simulink model "test_conv2drelu"  (R2017a)
settings: Solver=FixedStepDiscrete  StartTime=0.0  StopTime=1  FixedStep=1  RelTol=1e-3
undefined symbols (not defined in the file or in its folder): gray
libraries: ad_blocks x8, visionsources x1, visiongeotforms x1
settings Model: Creator=eruffaldi  LastModifiedBy=eruffaldi

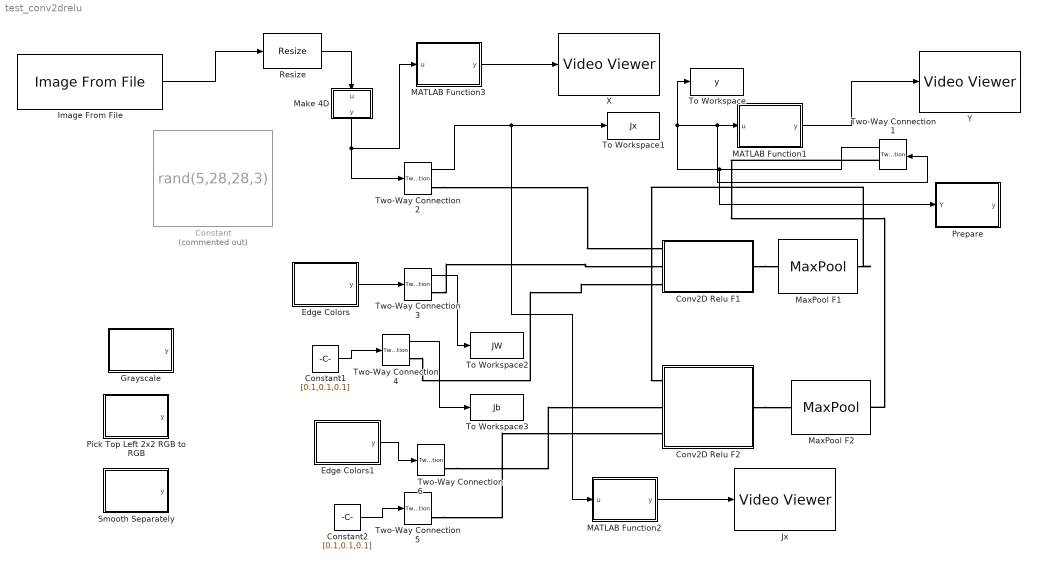
== system test_conv2drelu ==
  Constant : Constant  Commented=on  Value=rand(5,28,28,3)
  Constant1 : Constant  Value=[0.1,0.1,0.1]
  Constant2 : Constant  Value=[0.1,0.1,0.1]
  Conv2D Relu F1 : Subsystem
  Conv2D Relu F2 : Subsystem
  Edge Colors : MATLAB Function  TreatAsAtomicUnit=on
  Edge Colors1 : MATLAB Function  TreatAsAtomicUnit=on
  Grayscale : MATLAB Function  TreatAsAtomicUnit=on
  Image From File : visionsources/Image From File  Tag=vipblks_nd  FileName=peppers.png  imagePorts=One multidimensional signal  Ts=inf  ImageDataType=double  Signed=on  WordLength=16  sdImageDataType=uint(8)  FractionLengthMode=User-defined  FractionLength=15  OutPortLabels=R|G|B
      settings: SourceProductName=Computer Vision System Toolbox
  Jx : VideoViewer  colormapValue=gray(256)  FigPos=[1 894 1440 774]
  MATLAB Function1 : MATLAB Function  TreatAsAtomicUnit=on
  MATLAB Function2 : MATLAB Function  TreatAsAtomicUnit=on
  MATLAB Function3 : MATLAB Function  TreatAsAtomicUnit=on
  Make 4D : MATLAB Function  TreatAsAtomicUnit=on
  MaxPool F1 : ad_blocks/MaxPool  stride=[1,2,2,1]  ksize=[1,2,2,1]  padding=-1
  MaxPool F2 : ad_blocks/MaxPool  stride=[1,2,2,1]  ksize=[1,2,2,1]  padding=-1
  Pick Top Left 2x2 RGB to RGB : MATLAB Function  TreatAsAtomicUnit=on
  "Prepare " : MATLAB Function  TreatAsAtomicUnit=on
  Resize : visiongeotforms/Resize  specify=Number of output columns and preserve aspect ratio  rfactor=[200 150]  outCols=200  outRows=25  outRowsCols=[25 35]  interp_method=Bilinear  antialias=on  useROI=off  roiFlag=off  prodOutputMode=Binary point scaling  prodOutputWordLength=32  prodOutputFracLength=10  roundingMode=Nearest  overflowMode=on
      settings: SourceProductName=Computer Vision System Toolbox  SourceProductBaseCode=VP
  Smooth Separately : MATLAB Function  TreatAsAtomicUnit=on
  To Workspace : ToWorkspace  VariableName=y  SaveFormat=Timeseries  SampleTime=-1
  To Workspace1 : ToWorkspace  VariableName=Jx  SaveFormat=Timeseries  SampleTime=-1
  To Workspace2 : ToWorkspace  VariableName=JW  SaveFormat=Timeseries  SampleTime=-1
  To Workspace3 : ToWorkspace  VariableName=Jb  SaveFormat=Timeseries  SampleTime=-1
  Two-Way Connection{1..6} (6 alike) : TwoWayConnection
  X : VideoViewer  colormapValue=gray(256)  FigPos=[917 894 418 304]
  Y : VideoViewer  colormapValue=gray(256)  FigPos=[1 894 1440 774]
  wires:
  Two-Way Connection1/1 -> "Prepare "/1(Y), Two-Way Connection1/1, MATLAB Function1/1(u), To Workspace/1
  Two-Way Connection2/1 -> MATLAB Function2/1(u), To Workspace1/1
  Two-Way Connection3/1 -> To Workspace2/1
  Image From File/1 -> Resize/1
  Resize/1 -> Make 4D/1(u)
  Make 4D/1(y) -> MATLAB Function3/1(u), Two-Way Connection2/1
  MATLAB Function1/1(y) -> Y/1
  MATLAB Function3/1(y) -> X/1
  MATLAB Function2/1(y) -> Jx/1
  Edge Colors/1(y) -> Two-Way Connection3/1
  Constant1/1 -> Two-Way Connection4/1
  Two-Way Connection4/1 -> To Workspace3/1
  Edge Colors1/1(y) -> Two-Way Connection6/1
  Constant2/1 -> Two-Way Connection5/1
  connections:
  Two-Way Connection1/RConn1 -- MaxPool F2/RConn1
  Two-Way Connection2/RConn1 -- Conv2D Relu F1/LConn1
  Two-Way Connection4/RConn1 -- Conv2D Relu F1/LConn3
  Two-Way Connection3/RConn1 -- Conv2D Relu F1/LConn2
  Conv2D Relu F2/RConn1 -- MaxPool F2/LConn1
  Conv2D Relu F1/RConn1 -- MaxPool F1/LConn1
  MaxPool F1/RConn1 -- Conv2D Relu F2/LConn1
  Two-Way Connection5/RConn1 -- Conv2D Relu F2/LConn3
  Two-Way Connection6/RConn1 -- Conv2D Relu F2/LConn2

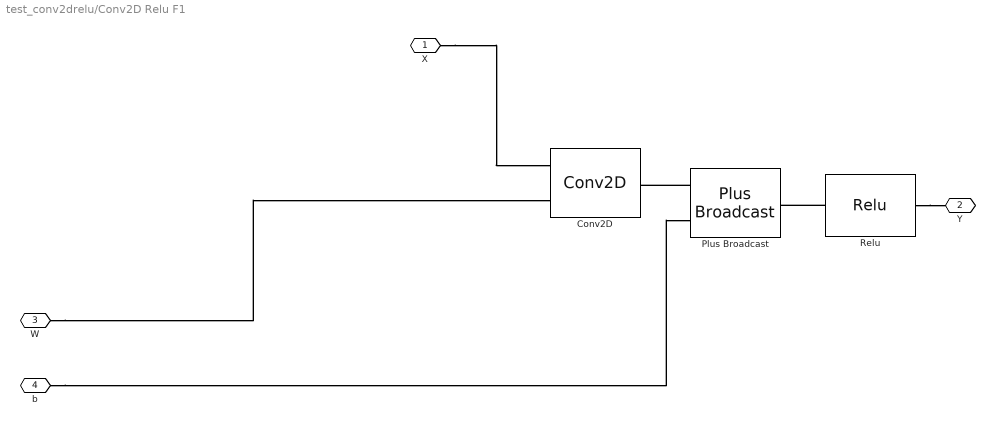
== system test_conv2drelu/Conv2D Relu F1 ==
  Conv2D : ad_blocks/Conv2D  stride=[1,2,2,1]  padding=-1
  Plus Broadcast : ad_blocks/Plus Broadcast
  Relu : ad_blocks/Relu
  X : PMIOPort  Port=1  Side=Left
  Y : PMIOPort  Port=2  Side=Right
  W : PMIOPort  Port=3  Side=Left
  b : PMIOPort  Port=4  Side=Left
  connections:
  Relu/LConn1 -- Plus Broadcast/RConn1
  Plus Broadcast/LConn1 -- Conv2D/RConn1
  Relu/RConn1 -- Y/RConn1
  b/RConn1 -- Plus Broadcast/LConn2
  X/RConn1 -- Conv2D/LConn1
  W/RConn1 -- Conv2D/LConn2

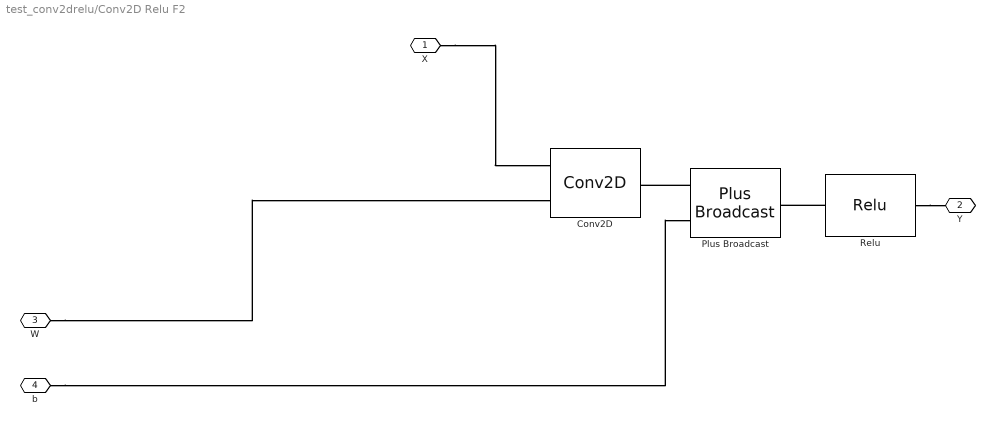
== system test_conv2drelu/Conv2D Relu F2 ==
  Conv2D : ad_blocks/Conv2D  stride=[1,2,2,1]  padding=-1
  Plus Broadcast : ad_blocks/Plus Broadcast
  Relu : ad_blocks/Relu
  X : PMIOPort  Port=1  Side=Left
  Y : PMIOPort  Port=2  Side=Right
  W : PMIOPort  Port=3  Side=Left
  b : PMIOPort  Port=4  Side=Left
  connections:
  W/RConn1 -- Conv2D/LConn2
  X/RConn1 -- Conv2D/LConn1
  b/RConn1 -- Plus Broadcast/LConn2
  Relu/RConn1 -- Y/RConn1
  Plus Broadcast/LConn1 -- Conv2D/RConn1
  Relu/LConn1 -- Plus Broadcast/RConn1

== matlab function test_conv2drelu/MATLAB Function1 ==
  data: y output; u input
function y = fcn(u)
y = squeeze(u(1,:,:,:));

== matlab function test_conv2drelu/Prepare  ==
  data: y output; Y input
function y = fcn(Y)

y = ones(size(Y));

== matlab function test_conv2drelu/Pick Top Left 2x2 RGB to RGB ==
  data: y output
function y = fcn()
y = zeros(2,2,3,3);

y(1,1,1,1) = 1;
y(1,1,2,2) = 1;
y(1,1,3,3) = 1;

== matlab function test_conv2drelu/MATLAB Function3 ==
  data: y output; u input
function y = fcn(u)
y = squeeze(u(1,:,:,:));

== matlab function test_conv2drelu/Smooth Separately ==
  data: y output
function y = fcn()
y = zeros(2,2,3,3);

y(:,:,1,1) = 1/4;
y(:,:,2,2) = 1/4;
y(:,:,3,3) = 1/4;

== matlab function test_conv2drelu/Make 4D ==
  data: y output; u input
function y = fcn(u)
y = reshape(u,[1,size(u)]);

== matlab function test_conv2drelu/Grayscale ==
  data: y output
function y = fcn()
y = zeros(2,2,3,1);
y(1,1,1,1) = 0.2989;
y(1,1,2,1) =  0.5870;
y(1,1,3,1) = 0.1140;

== matlab function test_conv2drelu/Edge Colors ==
  data: y output
function y = fcn()
y = zeros(3,3,3,3);

y(1,1,1,1) = -1;
y(2,1,1,1) =  -1;
y(3,1,1,1) = -1;

y(1,3,1,1) = 1;
y(2,3,1,1) =  1;
y(3,3,1,1) = 1;


y(1,1,1,2) = -1;
y(1,2,1,2) =  -1;
y(1,3,1,2) = -1;

y(3,1,1,2) = 1;
y(3,2,1,2) =  1;
y(3,3,1,2) = 1;

== matlab function test_conv2drelu/MATLAB Function2 ==
  data: y output; u input
function y = fcn(u)
y = squeeze(u(1,:,:,:));

== matlab function test_conv2drelu/Edge Colors1 ==
  data: y output
function y = fcn()
y = zeros(3,3,3,3);

y(1,1,1,1) = -1;
y(2,1,1,1) =  -1;
y(3,1,1,1) = -1;

y(1,3,1,1) = 1;
y(2,3,1,1) =  1;
y(3,3,1,1) = 1;


y(1,1,1,2) = -1;
y(1,2,1,2) =  -1;
y(1,3,1,2) = -1;

y(3,1,1,2) = 1;
y(3,2,1,2) =  1;
y(3,3,1,2) = 1;
